simulink model "inseguitore_manipolatore"  (R2024b)
settings: Solver=VariableStepAuto  StartTime=0.0  StopTime=100  RelTol=1e-3
values from neighbouring files (symbols this model uses):
  kd = K(:,3:4)    [regolatore_robot.m]
  kp = K(:,1:2)    [regolatore_robot.m]
  tau = 1    [regolatore_robot.m]
settings Model: Creator=Davide  LastModifiedBy=david
settings OptimizationCC: ReuseModelBlockBuffer=off
settings RTWCC: GPUComputeCapability=3.5

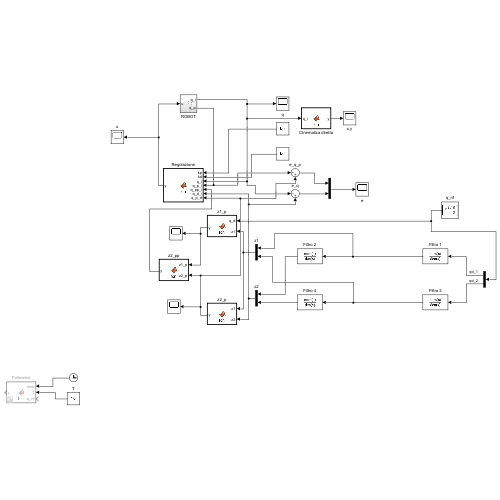
[thumbnail: Simulink's stored preview of the top-level diagram]
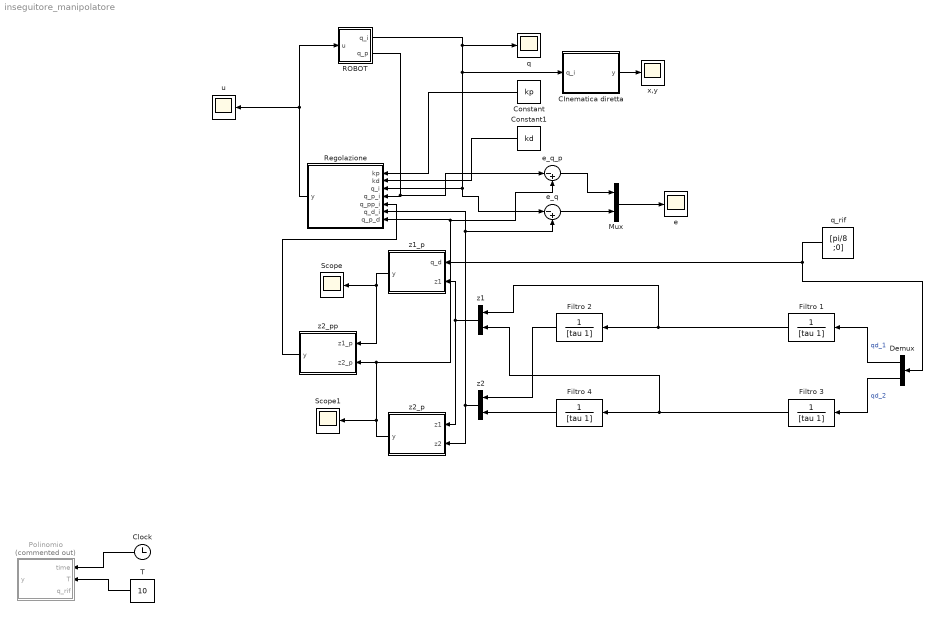
== system inseguitore_manipolatore ==
  CInematica diretta : MATLAB Function  TreatAsAtomicUnit=on
  Clock : Clock
  Constant : Constant  Value=kp  VectorParams1D=off
  Constant1 : Constant  Value=kd  VectorParams1D=off
  Demux : Demux  Outputs=2
  Filtro {1..4} (4 alike) : TransferFcn  Denominator=[tau 1]
  Mux : Mux  Inputs=2
  Polinomio : MATLAB Function  Commented=on  TreatAsAtomicUnit=on
  ROBOT : Subsystem
  Regolazione : MATLAB Function  TreatAsAtomicUnit=on
  Scope : Scope
  Scope1 : Scope
  T : Constant  Value=10  VectorParams1D=off
  e : Scope
  e_q : Sum  Inputs=|-+
  e_q_p : Sum  Inputs=|-+
  q : Scope
  q_rif : Constant  Value=[pi/8 ;0]  VectorParams1D=off
  u : Scope
  x,y : Scope
  z1 : Mux  Inputs=2
  z1_p : MATLAB Function  TreatAsAtomicUnit=on
  z2 : Mux  Inputs=2
  z2_p : MATLAB Function  TreatAsAtomicUnit=on
  z2_pp : MATLAB Function  TreatAsAtomicUnit=on
  wires:
  Regolazione/1(y) -> u/1, ROBOT/1(u)
  ROBOT/1(q_i) -> q/1, CInematica diretta/1(q_i), e_q/1, Regolazione/3(q_i)
  ROBOT/2(q_p) -> e_q_p/1, Regolazione/4(q_p_i)
  Constant/1 -> Regolazione/1(kp)
  Constant1/1 -> Regolazione/2(kd)
  CInematica diretta/1(y) -> x,y/1
  Clock/1 -> Polinomio/1(time)
  q_rif/1 -> Demux/1, z1_p/1(q_d)
  T/1 -> Polinomio/2(T)
  Demux/1 -> Filtro 1/1  "qd_1"
  Demux/2 -> Filtro 3/1  "qd_2"
  Filtro 1/1 -> Filtro 2/1, z1/1
  Filtro 3/1 -> Filtro 4/1, z1/2
  z1_p/1(y) -> z2_pp/1(z1_p), Scope/1
  z2_p/1(y) -> e_q_p/2, Regolazione/7(q_p_d), z2_pp/2(z2_p), Scope1/1
  z1/1 -> z2_p/1(z1), z1_p/2(z1)
  Filtro 2/1 -> z2/1
  z2/1 -> Regolazione/6(q_d_i), e_q/2, z2_p/2(z2)
  Filtro 4/1 -> z2/2
  z2_pp/1(y) -> Regolazione/5(q_pp_i)
  e_q/1 -> Mux/2
  Mux/1 -> e/1
  e_q_p/1 -> Mux/1

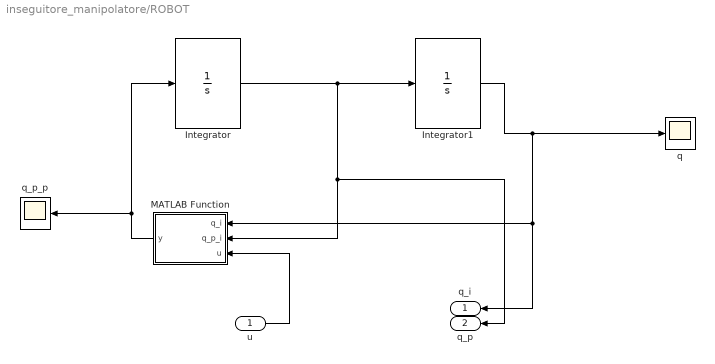
== system inseguitore_manipolatore/ROBOT ==
  u : Inport
  Integrator : Integrator  InitialCondition=[0;0]
  Integrator1 : Integrator  InitialCondition=[0;0]
  MATLAB Function : MATLAB Function  TreatAsAtomicUnit=on
  q : Scope
  q_p_p : Scope
  q_i : Outport
  q_p : Outport  Port=2
  wires:
  u/1 -> MATLAB Function/3(u)
  Integrator/1 -> q_p/1, MATLAB Function/2(q_p_i), Integrator1/1
  MATLAB Function/1(y) -> Integrator/1, q_p_p/1
  Integrator1/1 -> q_i/1, MATLAB Function/1(q_i), q/1

== matlab function inseguitore_manipolatore/ROBOT/MATLAB Function ==
  data: q_i input; q_p_i input; u input; y output
function y = fcn(q_i,q_p_i,u)


theta1 = 10.6125; 
theta2 = 0.85; 
theta3 = 2.25;
theta4 = 1.6;
theta5 = 80.9325;
theta6 = 14.7150;
q = q_i;
q_p = q_p_i;
v = u;
F1 = 15;
F2 = 10;

B = [theta1 + 2*theta3*q(2) theta2+theta3*cos(q(2)) ; ...
     theta2+theta3*cos(q(2)) theta4];
C = [-2*theta3*q_p(2)*sin(q(2))  -theta3*q_p(2)*sin(q(2)) ; ...
      theta3*q_p(1)*sin(q(2))              0              ];
g = [theta5*cos(q(1))+theta6*cos(q(1)+q(2)) ; theta6*cos(q(1)+q(2))];
F = [F1*q_p(1) ; F2*q_p(2)];

y = inv(B)*(v - g - F - C*q_p);

== matlab function inseguitore_manipolatore/Regolazione ==
  data: kp input; kd input; q_i input; q_p_i input; q_pp_i input; q_d_i input; y output; q_p_d input
function y = fcn(kp,kd,q_i,q_p_i,q_pp_i,q_d_i,q_p_d)


%k_p = 10*eye(2);
%k_d = 10*eye(2); 
theta1 = 10.6125; 
theta2 = 0.85; 
theta3 = 2.25;
theta4 = 1.6;
theta5 = 80.9325;
theta6 = 14.7150;
F1 = 15;
F2 = 10;
q = q_i;
q_p = q_p_i;
q_pp = q_pp_i;
q_d = q_d_i;
qp_d = q_p_d;

M =  [theta1 + 2*theta3*q(2) theta2+theta3*cos(q(2)) ; ...
     theta2+theta3*cos(q(2)) theta4];
C = [-2*theta3*q_p(2)*sin(q(2))  -theta3*q_p(2)*sin(q(2)) ; ...
      theta3*q_p(1)*sin(q(2))              0              ];
F = [F1*q_p(1)  F2*q_p(2)];
g = [theta5*cos(q(1))+theta6*cos(q(1)+q(2)) ; theta6*cos(q(1)+q(2))];


y = M*(q_pp + kp*(q_d-q) + kd*(qp_d-q_p)) + g + C*q_p + F*q_p ;

== matlab function inseguitore_manipolatore/Polinomio ==
  data: time input; T input; q_rif input; y output
function y = fcn(time,T,q_rif)


t = T;

q_r = q_rif;
a3 = (-2*q_r)/t;
a2 = (3*q_r)/t;
a1 = [0;0];
a0 = [0;0];
p_t = a3*time^3+a2*time^2+a1*time+a0;



y = p_t;

== matlab function inseguitore_manipolatore/CInematica diretta ==
  data: q_i input; y output
function y = fcn(q_i)

q = q_i;
l1 = 1.5;
l2 = 1;

%Estrazione posizione spazio operativo
y = [l1*cos(q(1))+l2*cos(q(2)) ; l1*sin(q(1))+l2*sin(q(2))];

== matlab function inseguitore_manipolatore/z1_p ==
  data: q_d input; z1 input; y output
function y = fcn(q_d,z1)


q = q_d;
tau = 1;
z1_p = (-1/tau)*z1+q;

y = z1_p;

== matlab function inseguitore_manipolatore/z2_p ==
  data: z1 input; z2 input; y output
function y = fcn(z1,z2)


tau = 1;
z2_p = (-1/tau)*z2+z1;

y = z2_p;

== matlab function inseguitore_manipolatore/z2_pp ==
  data: z1_p input; z2_p input; y output
function y = fcn(z1_p,z2_p)



tau = 1;
z2_pp = (-1/tau)*z2_p+z1_p;

y = z2_pp;
